simulink library "halin"  (R2021b)
settings: Solver=VariableStepAuto  StartTime=0.0  StopTime=10.0  RelTol=1e-3
undefined symbols (not defined in the file): TRUE
libraries: FVT_lib x100, hcu_lib x41
(part 2 of 10)

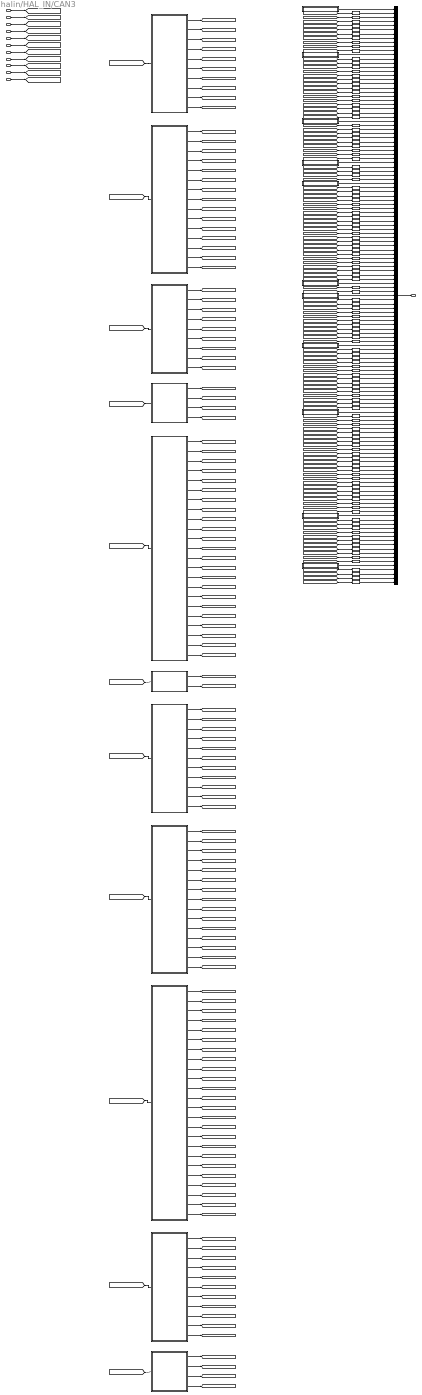
== system halin/HAL_IN/CAN3 ==
  DT_CAN3_SG_BMS1 : Inport
  DT_CAN3_SG_BMS3 : Inport  Port=2
  DT_CAN3_SG_BMS6 : Inport  Port=3
  DT_CAN3_SG_BMS8 : Inport  Port=4
  DT_CAN3_SG_CCU2 : Inport  Port=5
  DT_CAN3_SG_MCU_B_R1 : Inport  Port=6
  DT_CAN3_SG_Shifter1 : Inport  Port=7
  DT_CAN3_SG_BMS4 : Inport  Port=8
  DT_CAN3_SG_BMS5 : Inport  Port=9
  DT_CAN3_SG_CCU1 : Inport  Port=10
  DT_CAN3_SG_MCU_B_R2 : Inport  Port=11
  BMS1 : Subsystem
  BMS3 : Subsystem
  BMS4 : Subsystem
  BMS5 : Subsystem
  BMS6 : Subsystem
  BMS8 : Subsystem
  CCU1 : Subsystem
  CCU2 : Subsystem
  MCU_B_R1 : Subsystem
  MCU_B_R2 : Subsystem
  Shifter1 : Subsystem
  UnitConverter{,1,30..33,38..39,49..52,56..58,60..63,68,71,73..74,76,82,86..89,94,101,105,114..117,122..127} (42 alike) : DataTypeConversion  OutDataTypeStr=uint8
  UnitConverter{2..10,12..19,21..29,34..37,64..67,69..70,78..80,85,93,95..98,106..113,118..119} (55 alike) : DataTypeConversion  OutDataTypeStr=single
  UnitConverter{11,20,40..48,53..55,59,72,75,77,81,83..84,90..92,99..100,102..104} (29 alike) : DataTypeConversion  OutDataTypeStr=boolean
  UnitConverter120 : DataTypeConversion  OutDataTypeStr=uint16
  UnitConverter121 : DataTypeConversion  OutDataTypeStr=uint16
  VHAL_CANMsgInvalidBMS1_flg : Subsystem  AncestorBlock=FVT_lib/hal/MsgTimeoutJudge_CAN_AUTOSAR
      mask help: MeasumentTrigerEvent
      mask Display: fprintf('MsgTimeoutJudge_CAN\nAUTOSAR');
  VHAL_CANMsgInvalidBMS3_flg : Subsystem  AncestorBlock=FVT_lib/hal/MsgTimeoutJudge_CAN_AUTOSAR
      mask help: MeasumentTrigerEvent
      mask Display: fprintf('MsgTimeoutJudge_CAN\nAUTOSAR');
  VHAL_CANMsgInvalidBMS4_flg : Subsystem  AncestorBlock=FVT_lib/hal/MsgTimeoutJudge_CAN_AUTOSAR
      mask help: MeasumentTrigerEvent
      mask Display: fprintf('MsgTimeoutJudge_CAN\nAUTOSAR');
  VHAL_CANMsgInvalidBMS5_flg : Subsystem  AncestorBlock=FVT_lib/hal/MsgTimeoutJudge_CAN_AUTOSAR
      mask help: MeasumentTrigerEvent
      mask Display: fprintf('MsgTimeoutJudge_CAN\nAUTOSAR');
  VHAL_CANMsgInvalidBMS6_flg : Subsystem  AncestorBlock=FVT_lib/hal/MsgTimeoutJudge_CAN_AUTOSAR
      mask help: MeasumentTrigerEvent
      mask Display: fprintf('MsgTimeoutJudge_CAN\nAUTOSAR');
  VHAL_CANMsgInvalidBMS8_flg : Subsystem  AncestorBlock=FVT_lib/hal/MsgTimeoutJudge_CAN_AUTOSAR
      mask help: MeasumentTrigerEvent
      mask Display: fprintf('MsgTimeoutJudge_CAN\nAUTOSAR');
  VHAL_CANMsgInvalidCCU1_flg : Subsystem  AncestorBlock=FVT_lib/hal/MsgTimeoutJudge_CAN_AUTOSAR
      mask help: MeasumentTrigerEvent
      mask Display: fprintf('MsgTimeoutJudge_CAN\nAUTOSAR');
  VHAL_CANMsgInvalidCCU2_flg : Subsystem  AncestorBlock=FVT_lib/hal/MsgTimeoutJudge_CAN_AUTOSAR
      mask help: MeasumentTrigerEvent
      mask Display: fprintf('MsgTimeoutJudge_CAN\nAUTOSAR');
  VHAL_CANMsgInvalidMCUBR1_flg : Subsystem  AncestorBlock=FVT_lib/hal/MsgTimeoutJudge_CAN_AUTOSAR
      mask help: MeasumentTrigerEvent
      mask Display: fprintf('MsgTimeoutJudge_CAN\nAUTOSAR');
  VHAL_CANMsgInvalidMCUBR2_flg : Subsystem  AncestorBlock=FVT_lib/hal/MsgTimeoutJudge_CAN_AUTOSAR
      mask help: MeasumentTrigerEvent
      mask Display: fprintf('MsgTimeoutJudge_CAN\nAUTOSAR');
  VHAL_CANMsgInvalidShifter1_flg : Subsystem  AncestorBlock=FVT_lib/hal/MsgTimeoutJudge_CAN_AUTOSAR
      mask help: MeasumentTrigerEvent
      mask Display: fprintf('MsgTimeoutJudge_CAN\nAUTOSAR');
  bus_creator : BusCreator  Inputs=139
  HAL_CAN3_outputs : Outport
  wires:
  DT_CAN3_SG_BMS1/1 -> [DT_CAN3_SG_BMS1]
  DT_CAN3_SG_BMS3/1 -> [DT_CAN3_SG_BMS3]
  DT_CAN3_SG_BMS6/1 -> [DT_CAN3_SG_BMS6]
  DT_CAN3_SG_BMS8/1 -> [DT_CAN3_SG_BMS8]
  DT_CAN3_SG_CCU2/1 -> [DT_CAN3_SG_CCU2]
  DT_CAN3_SG_MCU_B_R1/1 -> [DT_CAN3_SG_MCU_B_R1]
  DT_CAN3_SG_Shifter1/1 -> [DT_CAN3_SG_Shifter1]
  DT_CAN3_SG_BMS4/1 -> [DT_CAN3_SG_BMS4]
  DT_CAN3_SG_BMS5/1 -> [DT_CAN3_SG_BMS5]
  DT_CAN3_SG_CCU1/1 -> [DT_CAN3_SG_CCU1]
  DT_CAN3_SG_MCU_B_R2/1 -> [DT_CAN3_SG_MCU_B_R2]
  [DT_CAN3_SG_BMS1] -> BMS1/1(DT_CAN3_SG_BMS1)
  [DT_CAN3_SG_BMS3] -> BMS3/1(DT_CAN3_SG_BMS3)
  [DT_CAN3_SG_BMS4] -> BMS4/1(DT_CAN3_SG_BMS4)
  [DT_CAN3_SG_BMS5] -> BMS5/1(DT_CAN3_SG_BMS5)
  [DT_CAN3_SG_BMS6] -> BMS6/1(DT_CAN3_SG_BMS6)
  [DT_CAN3_SG_BMS8] -> BMS8/1(DT_CAN3_SG_BMS8)
  [DT_CAN3_SG_CCU1] -> CCU1/1(DT_CAN3_SG_CCU1)
  [DT_CAN3_SG_CCU2] -> CCU2/1(DT_CAN3_SG_CCU2)
  [DT_CAN3_SG_MCU_B_R1] -> MCU_B_R1/1(DT_CAN3_SG_MCU_B_R1)
  [DT_CAN3_SG_MCU_B_R2] -> MCU_B_R2/1(DT_CAN3_SG_MCU_B_R2)
  [DT_CAN3_SG_Shifter1] -> Shifter1/1(DT_CAN3_SG_Shifter1)
  bus_creator/1 -> HAL_CAN3_outputs/1
  VHAL_CANMsgInvalidBMS1_flg/1(Out) -> bus_creator/1
  BMS1/1(VHAL_BMSChckSum1_enum) -> [VHAL_BMSChckSum1_enum]
  UnitConverter/1 -> bus_creator/2  "VHAL_BMSChckSum1_enum"
  [VHAL_BMSChckSum1_enum] -> UnitConverter/1
  BMS1/2(VHAL_BMSRolCnct1_enum) -> [VHAL_BMSRolCnct1_enum]
  UnitConverter1/1 -> bus_creator/3  "VHAL_BMSRolCnct1_enum"
  [VHAL_BMSRolCnct1_enum] -> UnitConverter1/1
  BMS1/3(VHAL_HVBPwrAvailChrg_kW) -> [VHAL_HVBPwrAvailChrg_kW]
  UnitConverter2/1 -> bus_creator/4  "VHAL_HVBPwrAvailChrg_kW"
  [VHAL_HVBPwrAvailChrg_kW] -> UnitConverter2/1
  BMS1/4(VHAL_HVBPwrAvailChrg30_kW) -> [VHAL_HVBPwrAvailChrg30_kW]
  UnitConverter3/1 -> bus_creator/5  "VHAL_HVBPwrAvailChrg30_kW"
  [VHAL_HVBPwrAvailChrg30_kW] -> UnitConverter3/1
  BMS1/5(VHAL_HVBPwrAvailChrg60_kW) -> [VHAL_HVBPwrAvailChrg60_kW]
  UnitConverter4/1 -> bus_creator/6  "VHAL_HVBPwrAvailChrg60_kW"
  [VHAL_HVBPwrAvailChrg60_kW] -> UnitConverter4/1
  BMS1/6(VHAL_HVBPwrAvailDchrg_kW) -> [VHAL_HVBPwrAvailDchrg_kW]
  UnitConverter5/1 -> bus_creator/7  "VHAL_HVBPwrAvailDchrg_kW"
  [VHAL_HVBPwrAvailDchrg_kW] -> UnitConverter5/1
  BMS1/7(VHAL_HVBPwrAvailDchrg30_kW) -> [VHAL_HVBPwrAvailDchrg30_kW]
  UnitConverter6/1 -> bus_creator/8  "VHAL_HVBPwrAvailDchrg30_kW"
  [VHAL_HVBPwrAvailDchrg30_kW] -> UnitConverter6/1
  BMS1/8(VHAL_HVBPwrAvailDchrg60_kW) -> [VHAL_HVBPwrAvailDchrg60_kW]
  UnitConverter7/1 -> bus_creator/9  "VHAL_HVBPwrAvailDchrg60_kW"
  [VHAL_HVBPwrAvailDchrg60_kW] -> UnitConverter7/1
  BMS1/9(VHAL_HVBattCurr_A) -> [VHAL_HVBattCurr_A]
  UnitConverter8/1 -> bus_creator/10  "VHAL_HVBattCurr_A"
  [VHAL_HVBattCurr_A] -> UnitConverter8/1
  BMS1/10(VHAL_HVBattVolt_V) -> [VHAL_HVBattVolt_V]
  UnitConverter9/1 -> bus_creator/11  "VHAL_HVBattVolt_V"
  [VHAL_HVBattVolt_V] -> UnitConverter9/1
  VHAL_CANMsgInvalidBMS3_flg/1(Out) -> bus_creator/12
  BMS3/1(VHAL_ACChrgCurrDis_A) -> [VHAL_ACChrgCurrDis_A]
  UnitConverter10/1 -> bus_creator/13  "VHAL_ACChrgCurrDis_A"
  [VHAL_ACChrgCurrDis_A] -> UnitConverter10/1
  BMS3/2(VHAL_FireDetErr_flg) -> [VHAL_FireDetErr_flg]
  UnitConverter11/1 -> bus_creator/14  "VHAL_FireDetErr_flg"
  [VHAL_FireDetErr_flg] -> UnitConverter11/1
  BMS3/3(VHAL_HVBChrgPwr_kWh) -> [VHAL_HVBChrgPwr_kWh]
  UnitConverter12/1 -> bus_creator/15  "VHAL_HVBChrgPwr_kWh"
  [VHAL_HVBChrgPwr_kWh] -> UnitConverter12/1
  BMS3/4(VHAL_HVBChrgPwrTotal_kWh) -> [VHAL_HVBChrgPwrTotal_kWh]
  UnitConverter13/1 -> bus_creator/16  "VHAL_HVBChrgPwrTotal_kWh"
  [VHAL_HVBChrgPwrTotal_kWh] -> UnitConverter13/1
  BMS3/5(VHAL_HVBDrvPwr_kWh) -> [VHAL_HVBDrvPwr_kWh]
  UnitConverter14/1 -> bus_creator/17  "VHAL_HVBDrvPwr_kWh"
  [VHAL_HVBDrvPwr_kWh] -> UnitConverter14/1
  BMS3/6(VHAL_HVBDrvPwrTotal_kWh) -> [VHAL_HVBDrvPwrTotal_kWh]
  UnitConverter15/1 -> bus_creator/18  "VHAL_HVBDrvPwrTotal_kWh"
  [VHAL_HVBDrvPwrTotal_kWh] -> UnitConverter15/1
  BMS3/7(VHAL_HVBFullChrgPwr_kWh) -> [VHAL_HVBFullChrgPwr_kWh]
  UnitConverter16/1 -> bus_creator/19  "VHAL_HVBFullChrgPwr_kWh"
  [VHAL_HVBFullChrgPwr_kWh] -> UnitConverter16/1
  BMS3/8(VHAL_HVBIsoImpedenceN_Megaohm) -> [VHAL_HVBIsoImpedenceN_Megaohm]
  UnitConverter17/1 -> bus_creator/20  "VHAL_HVBIsoImpedenceN_Megaohm"
  [VHAL_HVBIsoImpedenceN_Megaohm] -> UnitConverter17/1
  BMS3/9(VHAL_HVBIsoImpedenceP_Megaohm) -> [VHAL_HVBIsoImpedenceP_Megaohm]
  UnitConverter18/1 -> bus_creator/21  "VHAL_HVBIsoImpedenceP_Megaohm"
  [VHAL_HVBIsoImpedenceP_Megaohm] -> UnitConverter18/1
  BMS3/10(VHAL_HVBSOH_pct) -> [VHAL_HVBSOH_pct]
  UnitConverter19/1 -> bus_creator/22  "VHAL_HVBSOH_pct"
  [VHAL_HVBSOH_pct] -> UnitConverter19/1
  BMS3/11(VHAL_HVBattErr_flg) -> [VHAL_HVBattErr_flg]
  UnitConverter20/1 -> bus_creator/23  "VHAL_HVBattErr_flg"
  [VHAL_HVBattErr_flg] -> UnitConverter20/1
  BMS3/12(VHAL_HVBattPackVolt_V) -> [VHAL_HVBattPackVolt_V]
  UnitConverter21/1 -> bus_creator/24  "VHAL_HVBattPackVolt_V"
  [VHAL_HVBattPackVolt_V] -> UnitConverter21/1
  BMS3/13(VHAL_HVBattSOC_pct) -> [VHAL_HVBattSOC_pct]
  UnitConverter22/1 -> bus_creator/25  "VHAL_HVBattSOC_pct"
  [VHAL_HVBattSOC_pct] -> UnitConverter22/1
  BMS3/14(VHAL_HVBattSOCDis_pct) -> [VHAL_HVBattSOCDis_pct]
  UnitConverter23/1 -> bus_creator/26  "VHAL_HVBattSOCDis_pct"
  [VHAL_HVBattSOCDis_pct] -> UnitConverter23/1
  BMS3/15(VHAL_RemainChrgTime_min) -> [VHAL_RemainChrgTime_min]
  UnitConverter24/1 -> bus_creator/27  "VHAL_RemainChrgTime_min"
  [VHAL_RemainChrgTime_min] -> UnitConverter24/1
  VHAL_CANMsgInvalidBMS4_flg/1(Out) -> bus_creator/28
  BMS4/1(VHAL_CellTempAvg_C) -> [VHAL_CellTempAvg_C]
  UnitConverter25/1 -> bus_creator/29  "VHAL_CellTempAvg_C"
  [VHAL_CellTempAvg_C] -> UnitConverter25/1
  BMS4/2(VHAL_HVBCellVoltMax_mV) -> [VHAL_HVBCellVoltMax_mV]
  UnitConverter26/1 -> bus_creator/30  "VHAL_HVBCellVoltMax_mV"
  [VHAL_HVBCellVoltMax_mV] -> UnitConverter26/1
  BMS4/3(VHAL_HVBCellVoltMin_mV) -> [VHAL_HVBCellVoltMin_mV]
  UnitConverter27/1 -> bus_creator/31  "VHAL_HVBCellVoltMin_mV"
  [VHAL_HVBCellVoltMin_mV] -> UnitConverter27/1
  BMS4/4(VHAL_HVBMTempMax_C) -> [VHAL_HVBMTempMax_C]
  UnitConverter28/1 -> bus_creator/32  "VHAL_HVBMTempMax_C"
  [VHAL_HVBMTempMax_C] -> UnitConverter28/1
  BMS4/5(VHAL_HVBMTempMin_C) -> [VHAL_HVBMTempMin_C]
  UnitConverter29/1 -> bus_creator/33  "VHAL_HVBMTempMin_C"
  [VHAL_HVBMTempMin_C] -> UnitConverter29/1
  BMS4/6(VHAL_MaxCellTempNum_enum) -> [VHAL_MaxCellTempNum_enum]
  UnitConverter30/1 -> bus_creator/34  "VHAL_MaxCellTempNum_enum"
  [VHAL_MaxCellTempNum_enum] -> UnitConverter30/1
  BMS4/7(VHAL_MaxCellVoltNum_enum) -> [VHAL_MaxCellVoltNum_enum]
  UnitConverter31/1 -> bus_creator/35  "VHAL_MaxCellVoltNum_enum"
  [VHAL_MaxCellVoltNum_enum] -> UnitConverter31/1
  BMS4/8(VHAL_MinCellTempNum_enum) -> [VHAL_MinCellTempNum_enum]
  UnitConverter32/1 -> bus_creator/36  "VHAL_MinCellTempNum_enum"
  [VHAL_MinCellTempNum_enum] -> UnitConverter32/1
  BMS4/9(VHAL_MinCellVoltNum_enum) -> [VHAL_MinCellVoltNum_enum]
  UnitConverter33/1 -> bus_creator/37  "VHAL_MinCellVoltNum_enum"
  [VHAL_MinCellVoltNum_enum] -> UnitConverter33/1
  VHAL_CANMsgInvalidBMS5_flg/1(Out) -> bus_creator/38
  BMS5/1(VHAL_HVInVolt_V) -> [VHAL_HVInVolt_V]
  UnitConverter34/1 -> bus_creator/39  "VHAL_HVInVolt_V"
  [VHAL_HVInVolt_V] -> UnitConverter34/1
  BMS5/2(VHAL_LVBattDet12V_V) -> [VHAL_LVBattDet12V_V]
  UnitConverter35/1 -> bus_creator/40  "VHAL_LVBattDet12V_V"
  [VHAL_LVBattDet12V_V] -> UnitConverter35/1
  BMS5/3(VHAL_OBCDCCurLm_A) -> [VHAL_OBCDCCurLm_A]
  UnitConverter36/1 -> bus_creator/41  "VHAL_OBCDCCurLm_A"
  [VHAL_OBCDCCurLm_A] -> UnitConverter36/1
  BMS5/4(VHAL_OBCDCVoltLm_V) -> [VHAL_OBCDCVoltLm_V]
  UnitConverter37/1 -> bus_creator/42  "VHAL_OBCDCVoltLm_V"
  [VHAL_OBCDCVoltLm_V] -> UnitConverter37/1
  VHAL_CANMsgInvalidBMS6_flg/1(Out) -> bus_creator/43
  BMS6/1(VHAL_BMSChckSum_enum) -> [VHAL_BMSChckSum_enum]
  UnitConverter38/1 -> bus_creator/44  "VHAL_BMSChckSum_enum"
  [VHAL_BMSChckSum_enum] -> UnitConverter38/1
  BMS6/2(VHAL_BMSRolCnct_enum) -> [VHAL_BMSRolCnct_enum]
  UnitConverter39/1 -> bus_creator/45  "VHAL_BMSRolCnct_enum"
  [VHAL_BMSRolCnct_enum] -> UnitConverter39/1
  BMS6/3(VHAL_BMSREADY_flg) -> [VHAL_BMSREADY_flg]
  UnitConverter40/1 -> bus_creator/46  "VHAL_BMSREADY_flg"
  [VHAL_BMSREADY_flg] -> UnitConverter40/1
  BMS6/4(VHAL_BMSWarn1_flg) -> [VHAL_BMSWarn1_flg]
  UnitConverter41/1 -> bus_creator/47  "VHAL_BMSWarn1_flg"
  [VHAL_BMSWarn1_flg] -> UnitConverter41/1
  BMS6/5(VHAL_BMSWarn2_flg) -> [VHAL_BMSWarn2_flg]
  UnitConverter42/1 -> bus_creator/48  "VHAL_BMSWarn2_flg"
  [VHAL_BMSWarn2_flg] -> UnitConverter42/1
  BMS6/6(VHAL_BMSWarn3_flg) -> [VHAL_BMSWarn3_flg]
  UnitConverter43/1 -> bus_creator/49  "VHAL_BMSWarn3_flg"
  [VHAL_BMSWarn3_flg] -> UnitConverter43/1
  BMS6/7(VHAL_BMSWarn4_flg) -> [VHAL_BMSWarn4_flg]
  UnitConverter44/1 -> bus_creator/50  "VHAL_BMSWarn4_flg"
  [VHAL_BMSWarn4_flg] -> UnitConverter44/1
  BMS6/8(VHAL_BMSWarn5_flg) -> [VHAL_BMSWarn5_flg]
  UnitConverter45/1 -> bus_creator/51  "VHAL_BMSWarn5_flg"
  [VHAL_BMSWarn5_flg] -> UnitConverter45/1
  BMS6/9(VHAL_BMSWarn6_flg) -> [VHAL_BMSWarn6_flg]
  UnitConverter46/1 -> bus_creator/52  "VHAL_BMSWarn6_flg"
  [VHAL_BMSWarn6_flg] -> UnitConverter46/1
  BMS6/10(VHAL_BMSWarn7_flg) -> [VHAL_BMSWarn7_flg]
  UnitConverter47/1 -> bus_creator/53  "VHAL_BMSWarn7_flg"
  [VHAL_BMSWarn7_flg] -> UnitConverter47/1
  BMS6/11(VHAL_BMSWarn8_flg) -> [VHAL_BMSWarn8_flg]
  UnitConverter48/1 -> bus_creator/54  "VHAL_BMSWarn8_flg"
  [VHAL_BMSWarn8_flg] -> UnitConverter48/1
  BMS6/12(VHAL_ChrgPlugSta_enum) -> [VHAL_ChrgPlugSta_enum]
  UnitConverter49/1 -> bus_creator/55  "VHAL_ChrgPlugSta_enum"
  [VHAL_ChrgPlugSta_enum] -> UnitConverter49/1
  BMS6/13(VHAL_DisChrgPlugErr_enum) -> [VHAL_DisChrgPlugErr_enum]
  UnitConverter50/1 -> bus_creator/56  "VHAL_DisChrgPlugErr_enum"
  [VHAL_DisChrgPlugErr_enum] -> UnitConverter50/1
  BMS6/14(VHAL_ExtChrgSta_enum) -> [VHAL_ExtChrgSta_enum]
  UnitConverter51/1 -> bus_creator/57  "VHAL_ExtChrgSta_enum"
  [VHAL_ExtChrgSta_enum] -> UnitConverter51/1
  BMS6/15(VHAL_HVBChrgErr_enum) -> [VHAL_HVBChrgErr_enum]
  UnitConverter52/1 -> bus_creator/58  "VHAL_HVBChrgErr_enum"
  [VHAL_HVBChrgErr_enum] -> UnitConverter52/1
  BMS6/16(VHAL_HVBContactorSta_flg) -> [VHAL_HVBContactorSta_flg]
  UnitConverter53/1 -> bus_creator/59  "VHAL_HVBContactorSta_flg"
  [VHAL_HVBContactorSta_flg] -> UnitConverter53/1
  BMS6/17(VHAL_HVBHVILErr_flg) -> [VHAL_HVBHVILErr_flg]
  UnitConverter54/1 -> bus_creator/60  "VHAL_HVBHVILErr_flg"
  [VHAL_HVBHVILErr_flg] -> UnitConverter54/1
  BMS6/18(VHAL_HVBOvrTempErr_flg) -> [VHAL_HVBOvrTempErr_flg]
  UnitConverter55/1 -> bus_creator/61  "VHAL_HVBOvrTempErr_flg"
  [VHAL_HVBOvrTempErr_flg] -> UnitConverter55/1
  BMS6/19(VHAL_HVBOvrTempWarn_enum) -> [VHAL_HVBOvrTempWarn_enum]
  UnitConverter56/1 -> bus_creator/62  "VHAL_HVBOvrTempWarn_enum"
  [VHAL_HVBOvrTempWarn_enum] -> UnitConverter56/1
  BMS6/20(VHAL_HVBPreheatPrecoolSta_enum) -> [VHAL_HVBPreheatPrecoolSta_enum]
  UnitConverter57/1 -> bus_creator/63  "VHAL_HVBPreheatPrecoolSta_enum"
  [VHAL_HVBPreheatPrecoolSta_enum] -> UnitConverter57/1
  BMS6/21(VHAL_HVBattReady4Pre_enum) -> [VHAL_HVBattReady4Pre_enum]
  UnitConverter58/1 -> bus_creator/64  "VHAL_HVBattReady4Pre_enum"
  [VHAL_HVBattReady4Pre_enum] -> UnitConverter58/1
  BMS6/22(VHAL_HVILSta_flg) -> [VHAL_HVILSta_flg]
  UnitConverter59/1 -> bus_creator/65  "VHAL_HVILSta_flg"
  [VHAL_HVILSta_flg] -> UnitConverter59/1
  BMS6/23(VHAL_V2LSta_enum) -> [VHAL_V2LSta_enum]
  UnitConverter60/1 -> bus_creator/66  "VHAL_V2LSta_enum"
  [VHAL_V2LSta_enum] -> UnitConverter60/1
  VHAL_CANMsgInvalidBMS8_flg/1(Out) -> bus_creator/67
  BMS8/1(VHAL_MainRlyNegSta_enum) -> [VHAL_MainRlyNegSta_enum]
  UnitConverter61/1 -> bus_creator/68  "VHAL_MainRlyNegSta_enum"
  [VHAL_MainRlyNegSta_enum] -> UnitConverter61/1
  BMS8/2(VHAL_MainRlyPosSta_enum) -> [VHAL_MainRlyPosSta_enum]
  UnitConverter62/1 -> bus_creator/69  "VHAL_MainRlyPosSta_enum"
  [VHAL_MainRlyPosSta_enum] -> UnitConverter62/1
  VHAL_CANMsgInvalidCCU1_flg/1(Out) -> bus_creator/70
  CCU1/1(VHAL_CSCCU1_enum) -> [VHAL_CSCCU1_enum]
  UnitConverter63/1 -> bus_creator/71  "VHAL_CSCCU1_enum"
  [VHAL_CSCCU1_enum] -> UnitConverter63/1
  CCU1/2(VHAL_DCDCAuxCur_A) -> [VHAL_DCDCAuxCur_A]
  UnitConverter64/1 -> bus_creator/72  "VHAL_DCDCAuxCur_A"
  [VHAL_DCDCAuxCur_A] -> UnitConverter64/1
  CCU1/3(VHAL_DCDCAuxVolt_V) -> [VHAL_DCDCAuxVolt_V]
  UnitConverter65/1 -> bus_creator/73  "VHAL_DCDCAuxVolt_V"
  [VHAL_DCDCAuxVolt_V] -> UnitConverter65/1
  CCU1/4(VHAL_DCDCHVCur_A) -> [VHAL_DCDCHVCur_A]
  UnitConverter66/1 -> bus_creator/74  "VHAL_DCDCHVCur_A"
  [VHAL_DCDCHVCur_A] -> UnitConverter66/1
  CCU1/5(VHAL_DCDCInVoltInf_V) -> [VHAL_DCDCInVoltInf_V]
  UnitConverter67/1 -> bus_creator/75  "VHAL_DCDCInVoltInf_V"
  [VHAL_DCDCInVoltInf_V] -> UnitConverter67/1
  CCU1/6(VHAL_DCDCPreCompleted_enum) -> [VHAL_DCDCPreCompleted_enum]
  UnitConverter68/1 -> bus_creator/76  "VHAL_DCDCPreCompleted_enum"
  [VHAL_DCDCPreCompleted_enum] -> UnitConverter68/1
  CCU1/7(VHAL_OBCDCCurrInf_A) -> [VHAL_OBCDCCurrInf_A]
  UnitConverter69/1 -> bus_creator/77  "VHAL_OBCDCCurrInf_A"
  [VHAL_OBCDCCurrInf_A] -> UnitConverter69/1
  CCU1/8(VHAL_OBCDCVoltInf_V) -> [VHAL_OBCDCVoltInf_V]
  UnitConverter70/1 -> bus_creator/78  "VHAL_OBCDCVoltInf_V"
  [VHAL_OBCDCVoltInf_V] -> UnitConverter70/1
  CCU1/9(VHAL_OBCPreCompleted_enum) -> [VHAL_OBCPreCompleted_enum]
  UnitConverter71/1 -> bus_creator/79  "VHAL_OBCPreCompleted_enum"
  [VHAL_OBCPreCompleted_enum] -> UnitConverter71/1
  CCU1/10(VHAL_OBCWakeup4Plugin_flg) -> [VHAL_OBCWakeup4Plugin_flg]
  UnitConverter72/1 -> bus_creator/80  "VHAL_OBCWakeup4Plugin_flg"
  [VHAL_OBCWakeup4Plugin_flg] -> UnitConverter72/1
  CCU1/11(VHAL_RCCCU1_enum) -> [VHAL_RCCCU1_enum]
  UnitConverter73/1 -> bus_creator/81  "VHAL_RCCCU1_enum"
  [VHAL_RCCCU1_enum] -> UnitConverter73/1
  VHAL_CANMsgInvalidCCU2_flg/1(Out) -> bus_creator/82
  CCU2/1(VHAL_CSCCU2_enum) -> [VHAL_CSCCU2_enum]
  UnitConverter74/1 -> bus_creator/83  "VHAL_CSCCU2_enum"
  [VHAL_CSCCU2_enum] -> UnitConverter74/1
  CCU2/2(VHAL_DCDCEnaSta_flg) -> [VHAL_DCDCEnaSta_flg]
  UnitConverter75/1 -> bus_creator/84  "VHAL_DCDCEnaSta_flg"
  [VHAL_DCDCEnaSta_flg] -> UnitConverter75/1
  CCU2/3(VHAL_DCDCFaultSta_enum) -> [VHAL_DCDCFaultSta_enum]
  UnitConverter76/1 -> bus_creator/85  "VHAL_DCDCFaultSta_enum"
  [VHAL_DCDCFaultSta_enum] -> UnitConverter76/1
  CCU2/4(VHAL_DCDCReady4Pre_flg) -> [VHAL_DCDCReady4Pre_flg]
  UnitConverter77/1 -> bus_creator/86  "VHAL_DCDCReady4Pre_flg"
  [VHAL_DCDCReady4Pre_flg] -> UnitConverter77/1
  CCU2/5(VHAL_DCDCTemp_C) -> [VHAL_DCDCTemp_C]
  UnitConverter78/1 -> bus_creator/87  "VHAL_DCDCTemp_C"
  [VHAL_DCDCTemp_C] -> UnitConverter78/1
  CCU2/6(VHAL_OBCACCurrInf_A) -> [VHAL_OBCACCurrInf_A]
  UnitConverter79/1 -> bus_creator/88  "VHAL_OBCACCurrInf_A"
  [VHAL_OBCACCurrInf_A] -> UnitConverter79/1
  CCU2/7(VHAL_OBCACVoltInf_V) -> [VHAL_OBCACVoltInf_V]
  UnitConverter80/1 -> bus_creator/89  "VHAL_OBCACVoltInf_V"
  [VHAL_OBCACVoltInf_V] -> UnitConverter80/1
  CCU2/8(VHAL_OBCEnaSta_flg) -> [VHAL_OBCEnaSta_flg]
  UnitConverter81/1 -> bus_creator/90  "VHAL_OBCEnaSta_flg"
  [VHAL_OBCEnaSta_flg] -> UnitConverter81/1
  CCU2/9(VHAL_OBCFaultSta_enum) -> [VHAL_OBCFaultSta_enum]
  UnitConverter82/1 -> bus_creator/91  "VHAL_OBCFaultSta_enum"
  [VHAL_OBCFaultSta_enum] -> UnitConverter82/1
  CCU2/10(VHAL_OBCPluginSta_flg) -> [VHAL_OBCPluginSta_flg]
  UnitConverter83/1 -> bus_creator/92  "VHAL_OBCPluginSta_flg"
  [VHAL_OBCPluginSta_flg] -> UnitConverter83/1
  CCU2/11(VHAL_OBCReady4Pre_flg) -> [VHAL_OBCReady4Pre_flg]
  UnitConverter84/1 -> bus_creator/93  "VHAL_OBCReady4Pre_flg"
  [VHAL_OBCReady4Pre_flg] -> UnitConverter84/1
  CCU2/12(VHAL_OBCTemp_C) -> [VHAL_OBCTemp_C]
  UnitConverter85/1 -> bus_creator/94  "VHAL_OBCTemp_C"
  [VHAL_OBCTemp_C] -> UnitConverter85/1
  CCU2/13(VHAL_OBCV2LSta_enum) -> [VHAL_OBCV2LSta_enum]
  UnitConverter86/1 -> bus_creator/95  "VHAL_OBCV2LSta_enum"
  [VHAL_OBCV2LSta_enum] -> UnitConverter86/1
  CCU2/14(VHAL_OBCACCurLim_enum) -> [VHAL_OBCACCurLim_enum]
  UnitConverter87/1 -> bus_creator/96  "VHAL_OBCACCurLim_enum"
  [VHAL_OBCACCurLim_enum] -> UnitConverter87/1
  CCU2/15(VHAL_RCCCU2_enum) -> [VHAL_RCCCU2_enum]
  UnitConverter88/1 -> bus_creator/97  "VHAL_RCCCU2_enum"
  [VHAL_RCCCU2_enum] -> UnitConverter88/1
  VHAL_CANMsgInvalidMCUBR1_flg/1(Out) -> bus_creator/98
  MCU_B_R1/1(VHAL_MCUWarnR_enum) -> [VHAL_MCUWarnR_enum]
  UnitConverter89/1 -> bus_creator/99  "VHAL_MCUWarnR_enum"
  [VHAL_MCUWarnR_enum] -> UnitConverter89/1
  MCU_B_R1/2(VHAL_RrActvDmpDisabSta_flg) -> [VHAL_RrActvDmpDisabSta_flg]
  UnitConverter90/1 -> bus_creator/100  "VHAL_RrActvDmpDisabSta_flg"
  [VHAL_RrActvDmpDisabSta_flg] -> UnitConverter90/1
  MCU_B_R1/3(VHAL_RrEDUDrtSta_flg) -> [VHAL_RrEDUDrtSta_flg]
  UnitConverter91/1 -> bus_creator/101  "VHAL_RrEDUDrtSta_flg"
  [VHAL_RrEDUDrtSta_flg] -> UnitConverter91/1
  MCU_B_R1/4(VHAL_RrEDUOpratingSta_flg) -> [VHAL_RrEDUOpratingSta_flg]
  UnitConverter92/1 -> bus_creator/102  "VHAL_RrEDUOpratingSta_flg"
  [VHAL_RrEDUOpratingSta_flg] -> UnitConverter92/1
  MCU_B_R1/5(VHAL_RrEDURealTMTq_Nm) -> [VHAL_RrEDURealTMTq_Nm]
  UnitConverter93/1 -> bus_creator/103  "VHAL_RrEDURealTMTq_Nm"
  [VHAL_RrEDURealTMTq_Nm] -> UnitConverter93/1
  MCU_B_R1/6(VHAL_RrEDURotateDirction_enum) -> [VHAL_RrEDURotateDirction_enum]
  UnitConverter94/1 -> bus_creator/104  "VHAL_RrEDURotateDirction_enum"
  [VHAL_RrEDURotateDirction_enum] -> UnitConverter94/1
  MCU_B_R1/7(VHAL_RrEDUTqReqFbk_Nm) -> [VHAL_RrEDUTqReqFbk_Nm]
  UnitConverter95/1 -> bus_creator/105  "VHAL_RrEDUTqReqFbk_Nm"
  [VHAL_RrEDUTqReqFbk_Nm] -> UnitConverter95/1
  MCU_B_R1/8(VHAL_RrMCUBAT_V) -> [VHAL_RrMCUBAT_V]
  UnitConverter96/1 -> bus_creator/106  "VHAL_RrMCUBAT_V"
  [VHAL_RrMCUBAT_V] -> UnitConverter96/1
  MCU_B_R1/9(VHAL_RrMCUDCBusCurr_A) -> [VHAL_RrMCUDCBusCurr_A]
  UnitConverter97/1 -> bus_creator/107  "VHAL_RrMCUDCBusCurr_A"
  [VHAL_RrMCUDCBusCurr_A] -> UnitConverter97/1
  MCU_B_R1/10(VHAL_RrMCUDCBusVolt_V) -> [VHAL_RrMCUDCBusVolt_V]
  UnitConverter98/1 -> bus_creator/108  "VHAL_RrMCUDCBusVolt_V"
  [VHAL_RrMCUDCBusVolt_V] -> UnitConverter98/1
  MCU_B_R1/11(VHAL_RrMCUDischrgSta_flg) -> [VHAL_RrMCUDischrgSta_flg]
  UnitConverter99/1 -> bus_creator/109  "VHAL_RrMCUDischrgSta_flg"
  [VHAL_RrMCUDischrgSta_flg] -> UnitConverter99/1
  MCU_B_R1/12(VHAL_RrMCUEnaSta_flg) -> [VHAL_RrMCUEnaSta_flg]
  UnitConverter100/1 -> bus_creator/110  "VHAL_RrMCUEnaSta_flg"
  [VHAL_RrMCUEnaSta_flg] -> UnitConverter100/1
  MCU_B_R1/13(VHAL_RrMCUErr_enum) -> [VHAL_RrMCUErr_enum]
  UnitConverter101/1 -> bus_creator/111  "VHAL_RrMCUErr_enum"
  [VHAL_RrMCUErr_enum] -> UnitConverter101/1
  MCU_B_R1/14(VHAL_RrMCUIGNsta_flg) -> [VHAL_RrMCUIGNsta_flg]
  UnitConverter102/1 -> bus_creator/112  "VHAL_RrMCUIGNsta_flg"
  [VHAL_RrMCUIGNsta_flg] -> UnitConverter102/1
  MCU_B_R1/15(VHAL_RrMCUReady_flg) -> [VHAL_RrMCUReady_flg]
  UnitConverter103/1 -> bus_creator/113  "VHAL_RrMCUReady_flg"
  [VHAL_RrMCUReady_flg] -> UnitConverter103/1
  MCU_B_R1/16(VHAL_RrMCUReady4Pre_flg) -> [VHAL_RrMCUReady4Pre_flg]
  UnitConverter104/1 -> bus_creator/114  "VHAL_RrMCUReady4Pre_flg"
  [VHAL_RrMCUReady4Pre_flg] -> UnitConverter104/1
  MCU_B_R1/17(VHAL_RrMCUSysSta_enum) -> [VHAL_RrMCUSysSta_enum]
  UnitConverter105/1 -> bus_creator/115  "VHAL_RrMCUSysSta_enum"
  [VHAL_RrMCUSysSta_enum] -> UnitConverter105/1
  MCU_B_R1/18(VHAL_RrMCUTemp_C) -> [VHAL_RrMCUTemp_C]
  UnitConverter106/1 -> bus_creator/116  "VHAL_RrMCUTemp_C"
  [VHAL_RrMCUTemp_C] -> UnitConverter106/1
  MCU_B_R1/19(VHAL_RrMotorAvailTq_Nm) -> [VHAL_RrMotorAvailTq_Nm]
  UnitConverter107/1 -> bus_creator/117  "VHAL_RrMotorAvailTq_Nm"
  [VHAL_RrMotorAvailTq_Nm] -> UnitConverter107/1
  MCU_B_R1/20(VHAL_RrRegenAvailTq_Nm) -> [VHAL_RrRegenAvailTq_Nm]
  UnitConverter108/1 -> bus_creator/118  "VHAL_RrRegenAvailTq_Nm"
  [VHAL_RrRegenAvailTq_Nm] -> UnitConverter108/1
  MCU_B_R1/21(VHAL_RrTMSpd_rpm) -> [VHAL_RrTMSpd_rpm]
  UnitConverter109/1 -> bus_creator/119  "VHAL_RrTMSpd_rpm"
  [VHAL_RrTMSpd_rpm] -> UnitConverter109/1
  MCU_B_R1/22(VHAL_RrTMTemp_C) -> [VHAL_RrTMTemp_C]
  UnitConverter110/1 -> bus_creator/120  "VHAL_RrTMTemp_C"
  [VHAL_RrTMTemp_C] -> UnitConverter110/1
  MCU_B_R1/23(VHAL_RrTMid_A) -> [VHAL_RrTMid_A]
  UnitConverter111/1 -> bus_creator/121  "VHAL_RrTMid_A"
  [VHAL_RrTMid_A] -> UnitConverter111/1
  MCU_B_R1/24(VHAL_RrTMiq_A) -> [VHAL_RrTMiq_A]
  UnitConverter112/1 -> bus_creator/122  "VHAL_RrTMiq_A"
  [VHAL_RrTMiq_A] -> UnitConverter112/1
  VHAL_CANMsgInvalidMCUBR2_flg/1(Out) -> bus_creator/123
  MCU_B_R2/1(VHAL_RrCoolanttempReq_cnt) -> [VHAL_RrCoolanttempReq_cnt]
  UnitConverter113/1 -> bus_creator/124  "VHAL_RrCoolanttempReq_cnt"
  [VHAL_RrCoolanttempReq_cnt] -> UnitConverter113/1
  MCU_B_R2/2(VHAL_RrFailcode1_enum) -> [VHAL_RrFailcode1_enum]
  UnitConverter114/1 -> bus_creator/125  "VHAL_RrFailcode1_enum"
  [VHAL_RrFailcode1_enum] -> UnitConverter114/1
  MCU_B_R2/3(VHAL_RrFailcode2_enum) -> [VHAL_RrFailcode2_enum]
  UnitConverter115/1 -> bus_creator/126  "VHAL_RrFailcode2_enum"
  [VHAL_RrFailcode2_enum] -> UnitConverter115/1
  MCU_B_R2/4(VHAL_RrFailcodehistory1_enum) -> [VHAL_RrFailcodehistory1_enum]
  UnitConverter116/1 -> bus_creator/127  "VHAL_RrFailcodehistory1_enum"
  [VHAL_RrFailcodehistory1_enum] -> UnitConverter116/1
  MCU_B_R2/5(VHAL_RrFailcodehistory2_enum) -> [VHAL_RrFailcodehistory2_enum]
  UnitConverter117/1 -> bus_creator/128  "VHAL_RrFailcodehistory2_enum"
  [VHAL_RrFailcodehistory2_enum] -> UnitConverter117/1
  MCU_B_R2/6(VHAL_RrLLCTemp_C) -> [VHAL_RrLLCTemp_C]
  UnitConverter118/1 -> bus_creator/129  "VHAL_RrLLCTemp_C"
  [VHAL_RrLLCTemp_C] -> UnitConverter118/1
  MCU_B_R2/7(VHAL_RrLLCflowReq_Lpmin) -> [VHAL_RrLLCflowReq_Lpmin]
  UnitConverter119/1 -> bus_creator/130  "VHAL_RrLLCflowReq_Lpmin"
  [VHAL_RrLLCflowReq_Lpmin] -> UnitConverter119/1
  MCU_B_R2/8(VHAL_RrMCU3HWVer_enum) -> [VHAL_RrMCU3HWVer_enum]
  UnitConverter120/1 -> bus_creator/131  "VHAL_RrMCU3HWVer_enum"
  [VHAL_RrMCU3HWVer_enum] -> UnitConverter120/1
  MCU_B_R2/9(VHAL_RrMCU3SWVer_enum) -> [VHAL_RrMCU3SWVer_enum]
  UnitConverter121/1 -> bus_creator/132  "VHAL_RrMCU3SWVer_enum"
  [VHAL_RrMCU3SWVer_enum] -> UnitConverter121/1
  MCU_B_R2/10(VHAL_RrMCUTempWarn_enum) -> [VHAL_RrMCUTempWarn_enum]
  UnitConverter122/1 -> bus_creator/133  "VHAL_RrMCUTempWarn_enum"
  [VHAL_RrMCUTempWarn_enum] -> UnitConverter122/1
  MCU_B_R2/11(VHAL_RrTMTempWarn_enum) -> [VHAL_RrTMTempWarn_enum]
  UnitConverter123/1 -> bus_creator/134  "VHAL_RrTMTempWarn_enum"
  [VHAL_RrTMTempWarn_enum] -> UnitConverter123/1
  VHAL_CANMsgInvalidShifter1_flg/1(Out) -> bus_creator/135
  Shifter1/1(VHAL_ShifterCRC8_enum) -> [VHAL_ShifterCRC8_enum]
  UnitConverter124/1 -> bus_creator/136  "VHAL_ShifterCRC8_enum"
  [VHAL_ShifterCRC8_enum] -> UnitConverter124/1
  Shifter1/2(VHAL_ShifterFailsta_enum) -> [VHAL_ShifterFailsta_enum]
  UnitConverter125/1 -> bus_creator/137  "VHAL_ShifterFailsta_enum"
  [VHAL_ShifterFailsta_enum] -> UnitConverter125/1
  Shifter1/3(VHAL_ShifterHandleCmd_enum) -> [VHAL_ShifterHandleCmd_enum]
  UnitConverter126/1 -> bus_creator/138  "VHAL_ShifterHandleCmd_enum"
  [VHAL_ShifterHandleCmd_enum] -> UnitConverter126/1
  Shifter1/4(VHAL_ShifterRC_enum) -> [VHAL_ShifterRC_enum]
  UnitConverter127/1 -> bus_creator/139  "VHAL_ShifterRC_enum"
  [VHAL_ShifterRC_enum] -> UnitConverter127/1
